simulink model "fv_sim_linearized"  (R2021b)
settings: Solver=VariableStepAuto  StartTime=0.0  StopTime=10  RelTol=1e-3
values from neighbouring files (symbols this model uses):
  euler_angles_BfromN_0_deg = [0.017*0; 0.017*0; 0.017*0]    [run_simulation.m]
  EvB_BfromE_mps = [50; 0.00001; 10]    [run_simulation.m]
  ExE_BfromE_0_m = lla2ecef([lat_d, lon_d, ground_level_m + altitude_m])'    [run_simulation.m]
  g_mps2 = 9.81    [run_simulation.m]
  J_kgm2 = [J_xx, J_xy, J_xz ... (first row only)    [get_mass_props.m]
  ll_NfromE_deg = [lat_d, lon_d]    [run_simulation.m]
  m_kg = sum(cmg(:,1))    [get_mass_props.m]
  omega_BwrtI_rps_0 = omega_BwrtN_rps + omega_EwrtI_rps_0    [run_simulation.m]
  omega_BwrtN_rps = deg2rad(omega_BwrtN_dps)    [run_simulation.m]
  pitch_gain = pitch_kd    [lin_pure_damp.m]    (also in run_simulation.m = -200)
  re_m = 6378000    [run_simulation.m]
  thrust_N = 10    [run_simulation.m]
undefined symbols (not defined in the file or in its folder): aoa_gain, euler_angles_NfromB_0_rad, magnitude, quat_rate_IC
libraries: coordinate_transforms x14, aerolibconvert2 x5, aerolibutil x4, aerolibfltsims x4, simulink_extras x2, vrlib x2, sharedutil x1, aerolibanimutils x1, aerodynamics x1, kinematics x1, slpidlib x1, simulink x1
settings Model: Creator=Nikita  LastModifiedBy=Nikita
settings SolverCC: AlgebraicLoopSolver=TrustRegion
settings DebuggingCC: SFMachineParentedDataDiag=warning

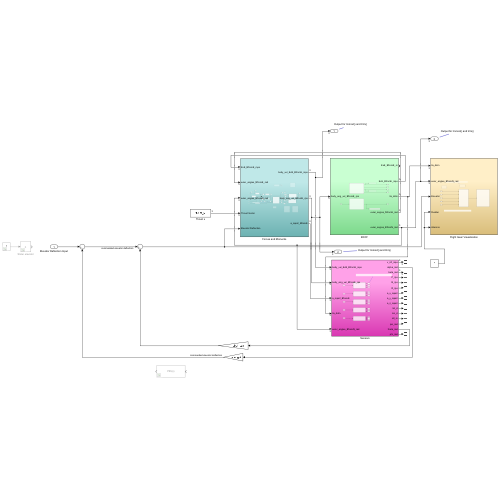
[thumbnail: Simulink's stored preview of the top-level diagram]
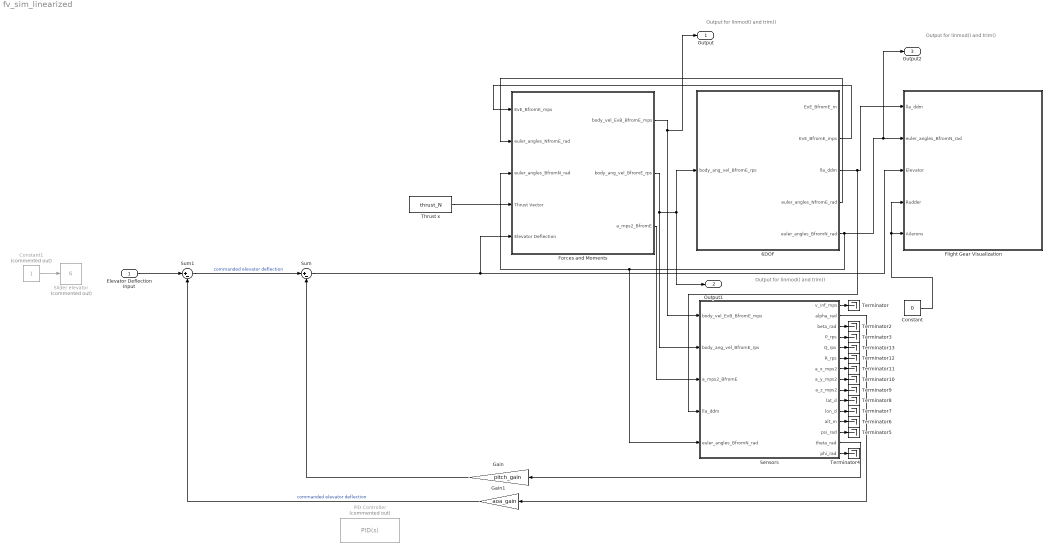
== system fv_sim_linearized ==
  note: Output for linmod() and trim()
  note: Output for linmod() and trim()
  note: Output for linmod() and trim()
  Elevator Deflection Input : Inport
  6DOF : Subsystem
  Constant : Constant  Value=0
  Constant1 : Constant  Commented=on
  Flight Gear Visualization : Subsystem
  Forces and Moments : Subsystem
  Gain : Gain  Gain=pitch_gain
  Gain1 : Gain  Gain=aoa_gain
  PID Controller : slpidlib/PID Controller  Commented=on  Controller=PID  Form=Parallel  TimeDomain=Continuous-time  UseExternalTs=off  SampleTime=-1  IntegratorMethod=Forward Euler  FilterMethod=Forward Euler  ControllerParametersSource=internal  P=-232.326301716838  I=-883.441178625002  D=-13.5750079022675  UseFilter=on  N=74490.174432495  TunerSelectOption=Transfer Function Based (PID Tuner App)  InitialConditionSource=internal  InitialConditionForIntegrator=0  InitialConditionForFilter=0  DifferentiatorICPrevScaledInput=0  ExternalReset=none  TrackingMode=off  Kt=1  LimitOutput=off  SatLimitsSource=internal  UpperSaturationLimit=inf  LowerSaturationLimit=-inf  LinearizeAsGain=on  AntiWindupMode=none  Kb=1  POutMin=[]  POutMax=[]  IOutMin=[]  IOutMax=[]  DOutMin=[]  DOutMax=[]  NOutMin=[]  NOutMax=[]  SumOutMin=[]  SumOutMax=[]  SaturationOutMin=[]  SaturationOutMax=[]  PParamMin=[]  PParamMax=[]  IParamMin=[]  IParamMax=[]  DParamMin=[]  DParamMax=[]  NParamMin=[]  NParamMax=[]  KbParamMin=[]  KbParamMax=[]  KtParamMin=[]  KtParamMax=[]  KbOutMin=[]  KbOutMax=[]  KtOutMin=[]  KtOutMax=[]  IntegratorOutMin=[]  IntegratorOutMax=[]  FilterOutMin=[]  FilterOutMax=[]  SumI1OutMin=[]  SumI1OutMax=[]  SumI2OutMin=[]  SumI2OutMax=[]  SumI3OutMin=[]  SumI3OutMax=[]  SumI4OutMin=[]  SumI4OutMax=[]  SumDOutMin=[]  SumDOutMax=[]  DifferentiatorOutMin=[]  DifferentiatorOutMax=[]  FilterDiffOutCoefMin=[]  FilterDiffOutCoefMax=[]  ReciprocalOutMin=[]  ReciprocalOutMax=[]  SumDenOutMin=[]  SumDenOutMax=[]  SumNumOutMin=[]  SumNumOutMax=[]  DivideOutMin=[]  DivideOutMax=[]  UdiffTsProdOutMin=[]  UdiffTsProdOutMax=[]  NTsProdOutMin=[]  NTsProdOutMax=[]  UintegralTsProdOutMin=[]  UintegralTsProdOutMax=[]  UngainTsProdOutMin=[]  UngainTsProdOutMax=[]  IntegratorContinuousStateAttributes=''  IntegratorStateMustResolveToSignalObject=off  IntegratorRTWStateStorageClass=Auto  FilterContinuousStateAttributes=''  FilterStateMustResolveToSignalObject=off  FilterRTWStateStorageClass=Auto  ParallelPVariant=InternalParameters  IdealPVariant=Disabled  IVariant=InternalParameters  DVariant=InternalParameters  IntegratorVariant=Continuous  SatVariant=Disabled  AWVariant=Passthrough  PCopyVariant=Disabled  TRVariant=Disabled  FdbkBlocksVariant=Forward  IdealPFdbkVariant=Disabled  SatFdbkVariant=Disabled  DerivativeFilterVariant=ContFilter  NVariant=InternalParameters  NCopyVariant=Disabled  FilterICVariant=InternalICsFilter  IntegratorICVariant=InternalICs  ExternalResetVariant=Disabled  TRSumVariant=Passthrough  SumFdbkVariant=Disabled  SumVariant=Sum_PID  TsampFilterVariant=InternalTs  TsampNgainVariant=Passthrough  TsampIntegralVariant=Passthrough  ExternalSaturationOutDataTypeStr=Inherit: Same as second input
  Sensors : Subsystem
  Slider elevator : simulink/Math Operations/Slider Gain  Commented=on  gain=6  low=-10  high=10
  Sum : Sum  Inputs=|+-
  Sum1 : Sum  Inputs=|+-
  Terminator{,2..13} (13 alike) : Terminator
  Thrust x : Constant  Value=thrust_N
  Output : Outport
  Output1 : Outport  Port=2
  Output2 : Outport  Port=3
  wires:
  6DOF/5(euler_angles_BfromN_rad) -> Sensors/5(euler_angles_BfromN_rad), Forces and Moments/3(euler_angles_BfromN_rad), Output2/1, Flight Gear Visualization/2(euler_angles_BfromN_rad)
  Forces and Moments/1(body_vel_EvB_BfromE_mps) -> Output/1, Sensors/1(body_vel_EvB_BfromE_mps)
  6DOF/3(lla_ddm) -> Flight Gear Visualization/1(lla_ddm), Sensors/4(lla_ddm)
  Constant/1 -> Flight Gear Visualization/5(Ailerons), Flight Gear Visualization/4(Rudder)
  6DOF/4(euler_angles_NfromE_rad) -> Forces and Moments/2(euler_angles_NfromE_rad)
  Forces and Moments/2(body_ang_vel_BfromE_rps) -> Sensors/2(body_ang_vel_BfromE_rps), 6DOF/1(body_ang_vel_BfromE_rps), Output1/1
  Forces and Moments/3(a_mps2_BfromE) -> Sensors/3(a_mps2_BfromE)
  Constant1/1 -> Slider elevator/1
  Sensors/14(theta_rad) -> Gain/1
  Sensors/1(v_inf_mps) -> Terminator/1
  Sensors/2(alpha_rad) -> Gain1/1
  Sensors/3(beta_rad) -> Terminator2/1
  Sensors/4(P_rps) -> Terminator3/1
  Sensors/15(phi_rad) -> Terminator4/1
  Sensors/13(psi_rad) -> Terminator5/1
  Sensors/12(alt_m) -> Terminator6/1
  Sensors/11(lon_d) -> Terminator7/1
  Sensors/10(lat_d) -> Terminator8/1
  Sensors/9(a_z_mps2) -> Terminator9/1
  Sensors/8(a_y_mps2) -> Terminator10/1
  Sensors/7(a_x_mps2) -> Terminator11/1
  Sensors/6(R_rps) -> Terminator12/1
  Sensors/5(Q_rps) -> Terminator13/1
  6DOF/2(EvE_BfromE_mps) -> Forces and Moments/1(EvE_BfromE_mps)
  Sum/1 -> Forces and Moments/5(Elevator Deflection), Flight Gear Visualization/3(Elevator)
  Gain/1 -> Sum/2
  Sum1/1 -> Sum/1  "commanded elevator deflection"
  Elevator Deflection Input/1 -> Sum1/1
  Gain1/1 -> Sum1/2  "commanded elevator deflection"
  Thrust x/1 -> Forces and Moments/4(Thrust Vector)

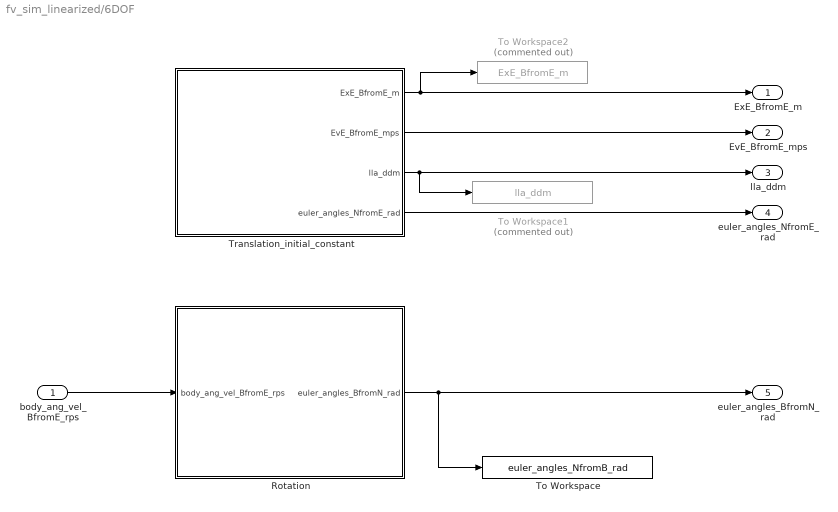
== system fv_sim_linearized/6DOF ==
  body_ang_vel_BfromE_rps : Inport
  Rotation : Subsystem
  To Workspace : ToWorkspace  VariableName=euler_angles_NfromB_rad  SampleTime=-1
  To Workspace1 : ToWorkspace  Commented=on  VariableName=lla_ddm  SampleTime=-1
  To Workspace2 : ToWorkspace  Commented=on  VariableName=ExE_BfromE_m  SampleTime=-1
  Translation_initial_constant : Subsystem
  ExE_BfromE_m : Outport
  EvE_BfromE_mps : Outport  Port=2
  lla_ddm : Outport  Port=3
  euler_angles_NfromE_rad : Outport  Port=4
  euler_angles_BfromN_rad : Outport  Port=5
  wires:
  Translation_initial_constant/3(lla_ddm) -> lla_ddm/1, To Workspace1/1
  Translation_initial_constant/1(ExE_BfromE_m) -> ExE_BfromE_m/1, To Workspace2/1
  Translation_initial_constant/2(EvE_BfromE_mps) -> EvE_BfromE_mps/1
  Rotation/1(euler_angles_BfromN_rad) -> euler_angles_BfromN_rad/1, To Workspace/1
  body_ang_vel_BfromE_rps/1 -> Rotation/1(body_ang_vel_BfromE_rps)
  Translation_initial_constant/4(euler_angles_NfromE_rad) -> euler_angles_NfromE_rad/1

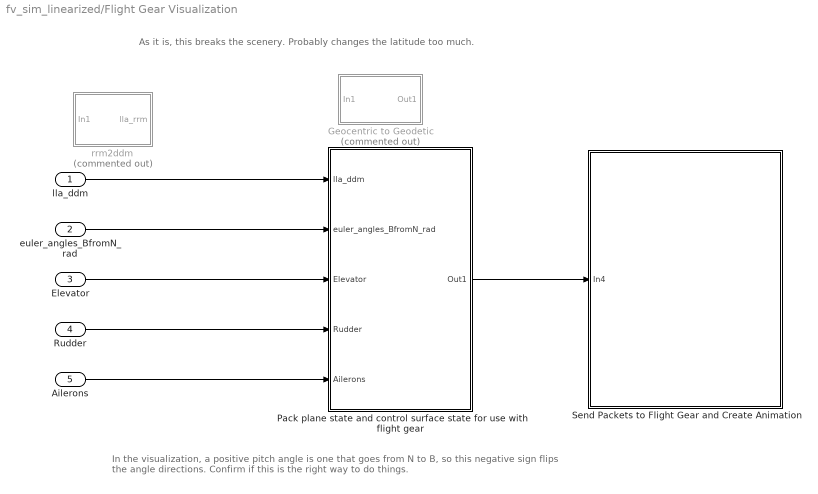
== system fv_sim_linearized/Flight Gear Visualization ==
  note: In the visualization, a positive pitch angle is one that goes from N to B, so this negative sign flips the angle directions. Confirm if this is the right way to do things.
  note: As it is, this breaks the scenery. Probably changes the latitude too much.
  lla_ddm : Inport
  euler_angles_BfromN_rad : Inport  Port=2
  Elevator : Inport  Port=3
  Rudder : Inport  Port=4
  Ailerons : Inport  Port=5
  Geocentric to Geodetic : Subsystem  Commented=on
  Pack plane state and control surface state for use with flight gear : Subsystem
  Send Packets to Flight Gear and Create Animation : Subsystem
  rrm2ddm : Subsystem  Commented=on
  wires:
  lla_ddm/1 -> Pack plane state and control surface state for use with flight gear/1(lla_ddm)
  Elevator/1 -> Pack plane state and control surface state for use with flight gear/3(Elevator)
  Rudder/1 -> Pack plane state and control surface state for use with flight gear/4(Rudder)
  Ailerons/1 -> Pack plane state and control surface state for use with flight gear/5(Ailerons)
  Pack plane state and control surface state for use with flight gear/1(Out1) -> Send Packets to Flight Gear and Create Animation/1(In4)
  euler_angles_BfromN_rad/1 -> Pack plane state and control surface state for use with flight gear/2(euler_angles_BfromN_rad)

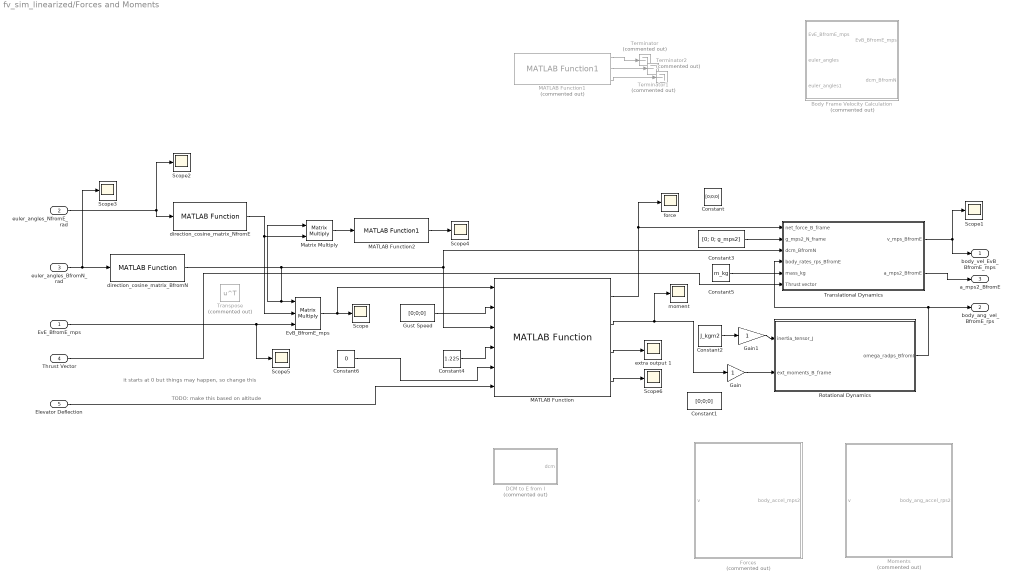
== system fv_sim_linearized/Forces and Moments ==
  note: it starts at 0 but things may happen, so change this
  note: TODO: make this based on altitude
  EvE_BfromE_mps : Inport
  euler_angles_NfromE_rad : Inport  Port=2
  euler_angles_BfromN_rad : Inport  Port=3
  Thrust Vector : Inport  Port=4
  Elevator Deflection : Inport  Port=5
  Body Frame Velocity Calculation : Subsystem  Commented=on
  Constant : Constant  Value=[0;0;0]
  Constant1 : Constant  Value=[0;0;0]
  Constant2 : Constant  Value=J_kgm2
  Constant3 : Constant  Value=[0; 0; g_mps2]
  Constant4 : Constant  Value=1.225
  Constant5 : Constant  Value=m_kg
  Constant6 : Constant  Value=0
  DCM to E from I : Subsystem  Commented=on
  EvB_BfromE_mps : Product  Inputs=3  Multiplication=Matrix(*)
  Forces : Subsystem  Commented=on
  Gain : Gain
  Gain1 : Gain
  Gust Speed : Constant  Value=[0;0;0]
  MATLAB Function : aerodynamics/MATLAB Function  SystemSampleTime=-1  VariantActivationTime=update diagram  Latency=0  AutoFrameSizeCalculation=off
  MATLAB Function1 : kinematics/MATLAB Function1  Commented=on  SystemSampleTime=-1  VariantActivationTime=update diagram  Latency=0  AutoFrameSizeCalculation=off
  MATLAB Function2 : coordinate_transforms/MATLAB Function1  SystemSampleTime=-1  VariantActivationTime=update diagram  Latency=0  AutoFrameSizeCalculation=off
  Matrix Multiply : Product  Multiplication=Matrix(*)
  Moments : Subsystem  Commented=on
  Rotational Dynamics : Subsystem
  Scope{,1..6} (7 alike) : Scope
  Terminator : Terminator  Commented=on
  Terminator1 : Terminator  Commented=on
  Terminator2 : Terminator  Commented=on
  Translational Dynamics : Subsystem
  Transpose : Math  Commented=on  Operator=transpose  SaturateOnIntegerOverflow=on
  direction_cosine_matrix_BfromN : coordinate_transforms/MATLAB Function  SystemSampleTime=-1  VariantActivationTime=update diagram  Latency=0  AutoFrameSizeCalculation=off
  direction_cosine_matrix_NfromE : coordinate_transforms/MATLAB Function  SystemSampleTime=-1  VariantActivationTime=update diagram  Latency=0  AutoFrameSizeCalculation=off
  extra output 1 : Scope
  force : Scope
  moment : Scope
  body_vel_EvB_BfromE_mps : Outport
  body_ang_vel_BfromE_rps : Outport  Port=2
  a_mps2_BfromE : Outport  Port=3
  wires:
  euler_angles_BfromN_rad/1 -> Scope3/1, direction_cosine_matrix_BfromN/1
  Translational Dynamics/1(v_mps_BfromE) -> body_vel_EvB_BfromE_mps/1, Scope1/1
  Rotational Dynamics/1(omega_radps_BfromI) -> body_ang_vel_BfromE_rps/1, Translational Dynamics/4(body_rates_rps_BfromE)
  Constant2/1 -> Gain1/1
  Constant3/1 -> Translational Dynamics/2(g_mps2_N_frame)
  Constant4/1 -> MATLAB Function/4
  Gust Speed/1 -> MATLAB Function/2
  MATLAB Function1/1 -> Terminator/1
  MATLAB Function1/2 -> Terminator1/1
  MATLAB Function1/3 -> Terminator2/1
  Constant5/1 -> Translational Dynamics/5(mass_kg)
  euler_angles_NfromE_rad/1 -> direction_cosine_matrix_NfromE/1, Scope2/1
  direction_cosine_matrix_NfromE/1 -> Matrix Multiply/2, EvB_BfromE_mps/2
  EvE_BfromE_mps/1 -> Scope5/1, EvB_BfromE_mps/3
  EvB_BfromE_mps/1 -> MATLAB Function/1, Scope/1
  MATLAB Function/1 -> force/1, Translational Dynamics/1(net_force_B_frame)
  MATLAB Function/2 -> moment/1, Gain/1
  MATLAB Function/3 -> extra output 1/1
  Gain/1 -> Rotational Dynamics/2(ext_moments_B_frame)
  Gain1/1 -> Rotational Dynamics/1(inertia_tensor_J)
  Constant6/1 -> MATLAB Function/5
  direction_cosine_matrix_BfromN/1 -> EvB_BfromE_mps/1, Matrix Multiply/1, MATLAB Function/3, Translational Dynamics/3(dcm_BfromN)
  MATLAB Function/4 -> Scope6/1
  Matrix Multiply/1 -> MATLAB Function2/1
  MATLAB Function2/1 -> Scope4/1
  Thrust Vector/1 -> Translational Dynamics/6(Thrust vector)
  Translational Dynamics/2(a_mps2_BfromE) -> a_mps2_BfromE/1
  Elevator Deflection/1 -> MATLAB Function/6

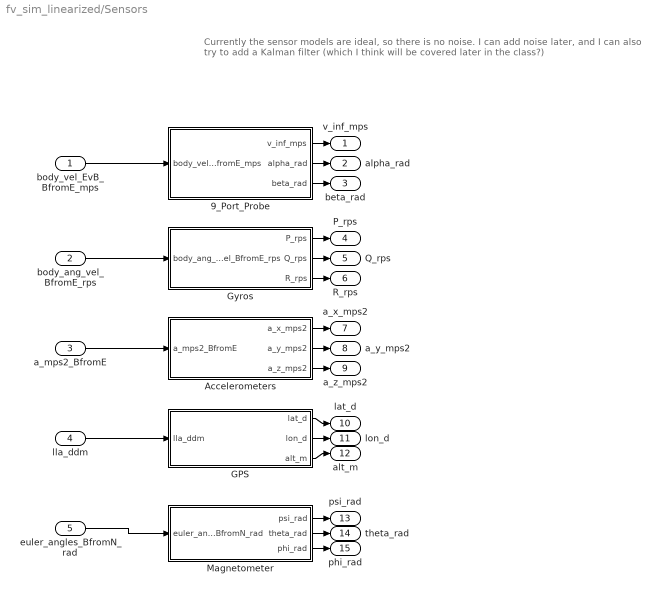
== system fv_sim_linearized/Sensors ==
  note: Currently the sensor models are ideal, so there is no noise. I can add noise later, and I can also try to add a Kalman filter (which I think will be covered later in the class?)
  body_vel_EvB_BfromE_mps : Inport
  body_ang_vel_BfromE_rps : Inport  Port=2
  a_mps2_BfromE : Inport  Port=3
  lla_ddm : Inport  Port=4
  euler_angles_BfromN_rad : Inport  Port=5
  9_Port_Probe : Subsystem
  Accelerometers : Subsystem
  GPS : Subsystem
  Gyros : Subsystem
  Magnetometer : Subsystem
  v_inf_mps : Outport
  alpha_rad : Outport  Port=2
  beta_rad : Outport  Port=3
  P_rps : Outport  Port=4
  Q_rps : Outport  Port=5
  R_rps : Outport  Port=6
  a_x_mps2 : Outport  Port=7
  a_y_mps2 : Outport  Port=8
  a_z_mps2 : Outport  Port=9
  lat_d : Outport  Port=10
  lon_d : Outport  Port=11
  alt_m : Outport  Port=12
  psi_rad : Outport  Port=13
  theta_rad : Outport  Port=14
  phi_rad : Outport  Port=15
  wires:
  9_Port_Probe/3(beta_rad) -> beta_rad/1
  body_vel_EvB_BfromE_mps/1 -> 9_Port_Probe/1(body_vel_EvB_BfromE_mps)
  body_ang_vel_BfromE_rps/1 -> Gyros/1(body_ang_vel_BfromE_rps)
  a_mps2_BfromE/1 -> Accelerometers/1(a_mps2_BfromE)
  Accelerometers/1(a_x_mps2) -> a_x_mps2/1
  Accelerometers/2(a_y_mps2) -> a_y_mps2/1
  9_Port_Probe/1(v_inf_mps) -> v_inf_mps/1
  9_Port_Probe/2(alpha_rad) -> alpha_rad/1
  Gyros/1(P_rps) -> P_rps/1
  Accelerometers/3(a_z_mps2) -> a_z_mps2/1
  Gyros/3(R_rps) -> R_rps/1
  Gyros/2(Q_rps) -> Q_rps/1
  lla_ddm/1 -> GPS/1(lla_ddm)
  GPS/1(lat_d) -> lat_d/1
  GPS/2(lon_d) -> lon_d/1
  GPS/3(alt_m) -> alt_m/1
  euler_angles_BfromN_rad/1 -> Magnetometer/1(euler_angles_BfromN_rad)
  Magnetometer/1(psi_rad) -> psi_rad/1
  Magnetometer/2(theta_rad) -> theta_rad/1
  Magnetometer/3(phi_rad) -> phi_rad/1

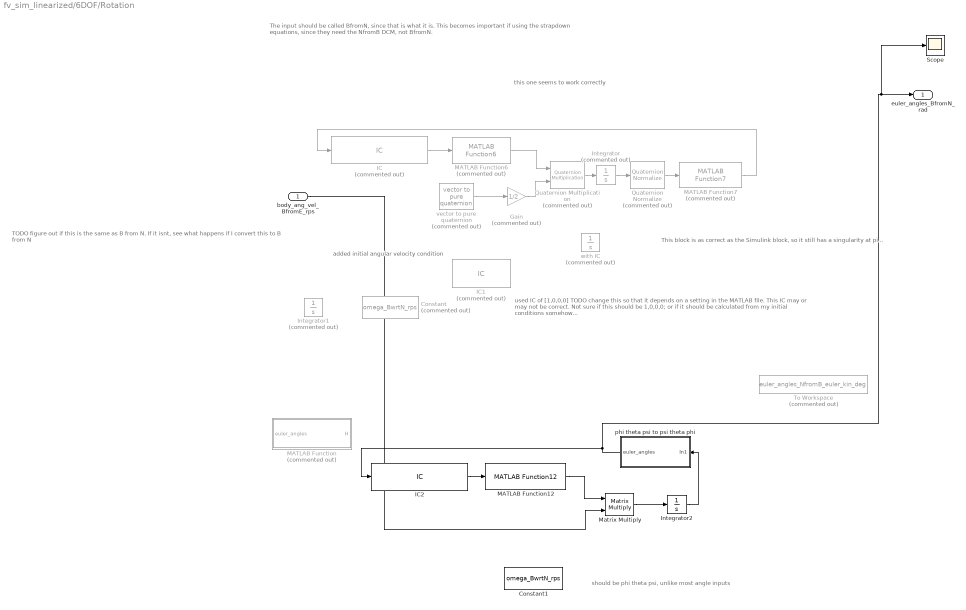
== system fv_sim_linearized/6DOF/Rotation ==
  note: TODO figure out if this is the same as B from N. If it isnt, see what happens if I convert this to B from N
  note: this one seems to work correctly
  note: This block is as correct as the Simulink block, so it still has a singularity at pi...
  note: The input should be called BfromN, since that is what it is.
      |
      | This becomes important if using the strapdown equations, since they need the NfromB DCM, not BfromN.
  note: used IC of [1,0,0,0]
      | TODO change this so that it depends on a setting in the MATLAB file. This IC may or may not be correct.
      | Not sure if this should be 1,0,0,0; or if it should be calculated from my initial conditions somehow...
  note: added initial angular velocity condition
  note: should be phi theta psi, unlike most angle inputs
  body_ang_vel_BfromE_rps : Inport
  Constant : Constant  Commented=on  Value=omega_BwrtN_rps
  Constant1 : Constant  Value=omega_BwrtN_rps
  Gain : Gain  Commented=on  Gain=1/2
  IC : InitialCondition  Commented=on  Value=euler_angles_NfromB_0_rad
  IC1 : InitialCondition  Commented=on  Value=omega_BwrtN_rps
  IC2 : InitialCondition  Value=euler_angles_BfromN_0_deg
  Integrator : Integrator  Commented=on  InitialCondition=[1;0;0;0]
  Integrator1 : Integrator  Commented=on  InitialCondition=omega_BwrtN_rps
  Integrator2 : Integrator  InitialCondition=euler_angles_BfromN_0_deg
  MATLAB Function : MATLAB Function  Commented=on  TreatAsAtomicUnit=on
  MATLAB Function12 : coordinate_transforms/MATLAB Function12  SystemSampleTime=-1  VariantActivationTime=update diagram  Latency=0  AutoFrameSizeCalculation=off
  MATLAB Function6 : coordinate_transforms/MATLAB Function6  Commented=on  SystemSampleTime=-1  VariantActivationTime=update diagram  Latency=0  AutoFrameSizeCalculation=off
  MATLAB Function7 : coordinate_transforms/MATLAB Function7  Commented=on  SystemSampleTime=-1  VariantActivationTime=update diagram  Latency=0  AutoFrameSizeCalculation=off
  Matrix Multiply : Product  Multiplication=Matrix(*)
  Quaternion Multiplication : aerolibutil/Quaternion Multiplication  Commented=on
  Quaternion Normalize : sharedutil/Quaternion Normalize  Commented=on  aMode=aMode
      settings: SourceProductBaseCode=AE,PW,DR,MT,UV,VE
  Scope : Scope
  To Workspace : ToWorkspace  Commented=on  VariableName=euler_angles_NfromB_euler_kin_deg  SampleTime=-1
  phi theta psi to psi theta phi : Subsystem
  vector to pure quaternion : coordinate_transforms/vector to pure quaternion  Commented=on  SystemSampleTime=-1  VariantActivationTime=update diagram  Latency=0  AutoFrameSizeCalculation=off
  with IC : Integrator  Commented=on  InitialCondition=quat_rate_IC
  euler_angles_BfromN_rad : Outport
  wires:
  Quaternion Multiplication/1 -> Integrator/1
  Gain/1 -> Quaternion Multiplication/2
  vector to pure quaternion/1 -> Gain/1
  Integrator/1 -> Quaternion Normalize/1
  IC/1 -> MATLAB Function6/1
  MATLAB Function6/1 -> Quaternion Multiplication/1
  Quaternion Normalize/1 -> MATLAB Function7/1
  MATLAB Function7/1 -> IC/1
  MATLAB Function12/1 -> Matrix Multiply/1
  Matrix Multiply/1 -> Integrator2/1
  Integrator2/1 -> phi theta psi to psi theta phi/1(In1)
  body_ang_vel_BfromE_rps/1 -> Matrix Multiply/2
  phi theta psi to psi theta phi/1(euler_angles) -> Scope/1, euler_angles_BfromN_rad/1, IC2/1
  IC2/1 -> MATLAB Function12/1

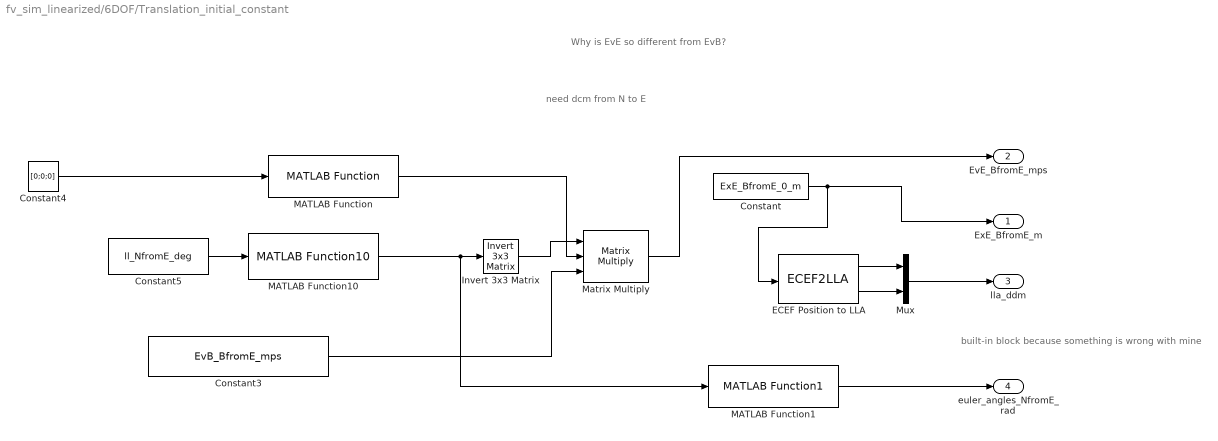
== system fv_sim_linearized/6DOF/Translation_initial_constant ==
  note: Why is EvE so different from EvB?
  note: built-in block because something is wrong with mine
  note: need dcm from N to E
  Constant : Constant  Value=ExE_BfromE_0_m
  Constant3 : Constant  Value=EvB_BfromE_mps
  Constant4 : Constant  Value=[0;0;0]
  Constant5 : Constant  Value=ll_NfromE_deg
  ECEF Position to LLA : ECEF2LLA
  Invert 3x3 Matrix : aerolibutil/Invert  3x3 Matrix
  MATLAB Function : coordinate_transforms/MATLAB Function  SystemSampleTime=-1  VariantActivationTime=update diagram  Latency=0  AutoFrameSizeCalculation=off
  MATLAB Function1 : coordinate_transforms/MATLAB Function1  SystemSampleTime=-1  VariantActivationTime=update diagram  Latency=0  AutoFrameSizeCalculation=off
  MATLAB Function10 : coordinate_transforms/MATLAB Function10  SystemSampleTime=-1  VariantActivationTime=update diagram  Latency=0  AutoFrameSizeCalculation=off
  Matrix Multiply : Product  Inputs=3  Multiplication=Matrix(*)
  Mux : Mux  Inputs=2
  ExE_BfromE_m : Outport
  EvE_BfromE_mps : Outport  Port=2
  lla_ddm : Outport  Port=3
  euler_angles_NfromE_rad : Outport  Port=4
  wires:
  Invert 3x3 Matrix/1 -> Matrix Multiply/1
  Matrix Multiply/1 -> EvE_BfromE_mps/1
  Constant5/1 -> MATLAB Function10/1
  MATLAB Function10/1 -> Invert 3x3 Matrix/1, MATLAB Function1/1
  MATLAB Function1/1 -> euler_angles_NfromE_rad/1
  Constant4/1 -> MATLAB Function/1
  Constant3/1 -> Matrix Multiply/3
  ECEF Position to LLA/2 -> Mux/2
  Mux/1 -> lla_ddm/1
  ECEF Position to LLA/1 -> Mux/1
  MATLAB Function/1 -> Matrix Multiply/2
  Constant/1 -> ECEF Position to LLA/1, ExE_BfromE_m/1

== system fv_sim_linearized/Flight Gear Visualization/Geocentric to Geodetic ==
  In1 : Inport
  Constant1 : Constant  Value=re_m
  Demux : Demux  Outputs=3
  Geocentric to Geodetic Latitude : Geoc2Geod
  Mux2 : Mux  Inputs=3
  Sum : Sum  Inputs=|++
  Out1 : Outport
  wires:
  Constant1/1 -> Sum/2
  Geocentric to Geodetic Latitude/1 -> Mux2/1
  Demux/3 -> Mux2/3, Sum/1
  Demux/1 -> Geocentric to Geodetic Latitude/1
  Sum/1 -> Geocentric to Geodetic Latitude/2
  Demux/2 -> Mux2/2
  In1/1 -> Demux/1
  Mux2/1 -> Out1/1

== system fv_sim_linearized/Flight Gear Visualization/Pack plane state and control surface state for use with flight gear ==
  note: try without this at some point, it seems to change the output data
  note: state (lla_ddm and euler angles in ECEF)
  lla_ddm : Inport
  euler_angles_BfromN_rad : Inport  Port=2
  Elevator : Inport  Port=3
  Rudder : Inport  Port=4
  Ailerons : Inport  Port=5
  Mux : Mux  Inputs=2
  Mux3 : Mux
  Rate Transition : RateTransition  Integrity=off  OutPortSampleTime=1/30
  Out1 : Outport
  wires:
  Ailerons/1 -> Mux3/4
  euler_angles_BfromN_rad/1 -> Mux/2
  Rudder/1 -> Mux3/3
  Mux/1 -> Mux3/1
  Mux3/1 -> Rate Transition/1
  Elevator/1 -> Mux3/2
  Rate Transition/1 -> Out1/1
  lla_ddm/1 -> Mux/1

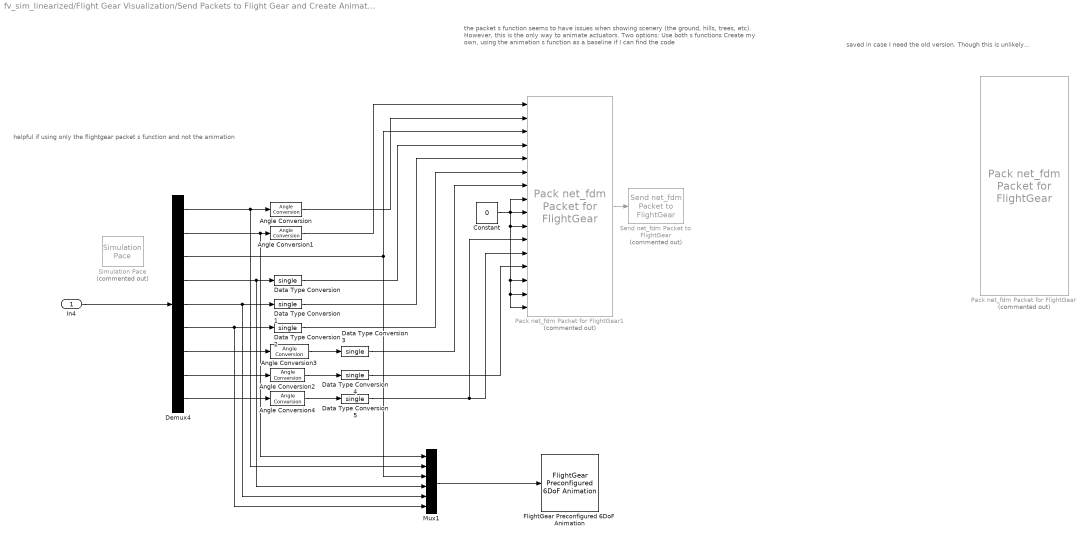
== system fv_sim_linearized/Flight Gear Visualization/Send Packets to Flight Gear and Create Animation ==
  note: the packet s function seems to have issues when showing scenery (the ground, hills, trees, etc). However, this is the only way to animate actuators. Two options:
      | Use both s functions
      | Create my own, using the animation s function as a baseline if I can find the code
  note: saved in case I need the old version. Though this is unlikely...
  note: helpful if using only the flightgear packet s function and not the animation
  In4 : Inport
  Angle Conversion : aerolibconvert2/Angle Conversion  IU=deg  OU=rad
  Angle Conversion1 : aerolibconvert2/Angle Conversion  IU=deg  OU=rad
  Angle Conversion2 : aerolibconvert2/Angle Conversion  IU=rad  OU=deg
  Angle Conversion3 : aerolibconvert2/Angle Conversion  IU=rad  OU=deg
  Angle Conversion4 : aerolibconvert2/Angle Conversion  IU=rad  OU=deg
  Constant : Constant  Value=0
  Data Type Conversion{,1..5} (6 alike) : DataTypeConversion  OutDataTypeStr=single
  Demux4 : Demux  Outputs=9
  FlightGear Preconfigured 6DoF Animation : aerolibfltsims/FlightGear Preconfigured 6DoF Animation  xFlightGearVersion=v2019.1  DestinationIpAddress=127.0.0.1  DestinationPort=5502  SampleTime=1/30  packetVersion=24
  Mux1 : Mux  Inputs=6
  Pack net_fdm Packet for FlightGear : aerolibfltsims/Pack net_fdm Packet for FlightGear  Commented=on  FlightGearVersion=v2019.1  ShowPositionAttitudeInputs=on  ShowVelocityAccelerationInputs=off  ShowControlSurfacePositionInputs=on  ShowEngineFuelInputs=off  ShowLandingGearInputs=off  ShowEnvironmentInputs=off  SampleTime=1/30  packetVersion=24
      settings: SourceProductBaseCode=AE
  Pack net_fdm Packet for FlightGear1 : aerolibfltsims/Pack net_fdm Packet for FlightGear  Commented=on  FlightGearVersion=v2019.1  ShowPositionAttitudeInputs=on  ShowVelocityAccelerationInputs=off  ShowControlSurfacePositionInputs=on  ShowEngineFuelInputs=off  ShowLandingGearInputs=off  ShowEnvironmentInputs=off  SampleTime=1/30  packetVersion=24
      settings: SourceProductBaseCode=AE
  Send net_fdm Packet to FlightGear : aerolibfltsims/Send net_fdm Packet to FlightGear  Commented=on  DestinationIpAddress=127.0.0.1  DestinationPort=5502  LocalIpPort=-1  varLen=off  SampleTime=1/30
      settings: SourceProductBaseCode=AE
  Simulation Pace : aerolibanimutils/Simulation Pace  Commented=on  SimulationPace=1  SleepMode=MATLAB Thread  OutputPaceError=off  SampleTime=1/30
      settings: AttributesFormatString=%<SimulationPace> sec/sec
  wires:
  Data Type Conversion2/1 -> Pack net_fdm Packet for FlightGear1/6
  Mux1/1 -> FlightGear Preconfigured 6DoF Animation/1
  Angle Conversion1/1 -> Pack net_fdm Packet for FlightGear1/1
  Angle Conversion2/1 -> Data Type Conversion4/1
  Demux4/9 -> Angle Conversion4/1
  Angle Conversion3/1 -> Data Type Conversion3/1
  Demux4/3 -> Pack net_fdm Packet for FlightGear1/3, Mux1/3
  Demux4/4 -> Mux1/4, Data Type Conversion/1
  Data Type Conversion5/1 -> Pack net_fdm Packet for FlightGear1/12, Pack net_fdm Packet for FlightGear1/11
  Angle Conversion/1 -> Pack net_fdm Packet for FlightGear1/2
  In4/1 -> Demux4/1
  Demux4/6 -> Mux1/6, Data Type Conversion2/1
  Angle Conversion4/1 -> Data Type Conversion5/1
  Constant/1 -> Pack net_fdm Packet for FlightGear1/9, Pack net_fdm Packet for FlightGear1/8, Pack net_fdm Packet for FlightGear1/16, Pack net_fdm Packet for FlightGear1/15, Pack net_fdm Packet for FlightGear1/14, Pack net_fdm Packet for FlightGear1/10
  Data Type Conversion1/1 -> Pack net_fdm Packet for FlightGear1/5
  Data Type Conversion3/1 -> Pack net_fdm Packet for FlightGear1/7
  Data Type Conversion/1 -> Pack net_fdm Packet for FlightGear1/4
  Demux4/5 -> Mux1/5, Data Type Conversion1/1
  Demux4/1 -> Mux1/2, Angle Conversion/1
  Demux4/2 -> Mux1/1, Angle Conversion1/1
  Demux4/8 -> Angle Conversion2/1
  Data Type Conversion4/1 -> Pack net_fdm Packet for FlightGear1/13
  Demux4/7 -> Angle Conversion3/1
  Pack net_fdm Packet for FlightGear1/1 -> Send net_fdm Packet to FlightGear/1

== system fv_sim_linearized/Flight Gear Visualization/rrm2ddm ==
  In1 : Inport
  Demux : Demux  Outputs=3
  Mux1 : Mux  Inputs=3
  Radians to Degrees : simulink_extras/Transformations/Radians to Degrees
  Radians to Degrees1 : simulink_extras/Transformations/Radians to Degrees
  lla_rrm : Outport
  wires:
  Demux/1 -> Radians to Degrees/1
  Radians to Degrees/1 -> Mux1/1
  Mux1/1 -> lla_rrm/1
  Demux/2 -> Radians to Degrees1/1
  Demux/3 -> Mux1/3
  Radians to Degrees1/1 -> Mux1/2
  In1/1 -> Demux/1

== system fv_sim_linearized/Forces and Moments/Body Frame Velocity Calculation ==
  note: converting EvE velocity to EvB for drag calculation
  EvE_BfromE_mps : Inport
  euler_angles : Inport  Port=2
  euler_angles1 : Inport  Port=3
  Matrix Multiply : Product  Inputs=3  Multiplication=Matrix(*)
  dcm_NfromE : coordinate_transforms/MATLAB Function  SystemSampleTime=-1  VariantActivationTime=update diagram  Latency=0  AutoFrameSizeCalculation=off
  direction_cosine_matrix_BfromN : coordinate_transforms/MATLAB Function  SystemSampleTime=-1  VariantActivationTime=update diagram  Latency=0  AutoFrameSizeCalculation=off
  EvB_BfromE_mps : Outport
  dcm_BfromN : Outport  Port=2
  wires:
  Matrix Multiply/1 -> EvB_BfromE_mps/1
  EvE_BfromE_mps/1 -> Matrix Multiply/3
  direction_cosine_matrix_BfromN/1 -> dcm_BfromN/1, Matrix Multiply/1
  dcm_NfromE/1 -> Matrix Multiply/2
  euler_angles/1 -> direction_cosine_matrix_BfromN/1
  euler_angles1/1 -> dcm_NfromE/1

== system fv_sim_linearized/Forces and Moments/DCM to E from I ==
  note: angles to E from I
  Clock : Clock
  MATLAB Function : coordinate_transforms/MATLAB Function  SystemSampleTime=-1  Latency=0  AutoFrameSizeCalculation=off
  Product : Product
  rotation of Earth : Constant  Value=omega_BwrtI_rps_0
  dcm : Outport
  wires:
  Clock/1 -> Product/1
  Product/1 -> MATLAB Function/1
  rotation of Earth/1 -> Product/2
  MATLAB Function/1 -> dcm/1

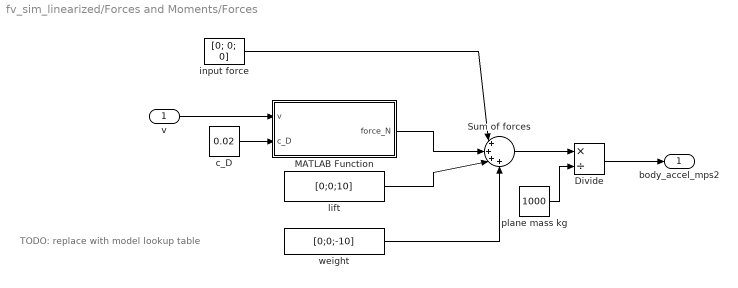
== system fv_sim_linearized/Forces and Moments/Forces ==
  note: TODO: replace with model lookup table
  v : Inport
  Divide : Product  Inputs=*/
  MATLAB Function : MATLAB Function  TreatAsAtomicUnit=on
  Sum of forces : Sum  Inputs=|++++
  c_D : Constant  Value=0.02
  input force : Constant  Value=[0; 0; 0]
  lift : Constant  Value=[0;0;10]
  plane mass kg : Constant  Value=1000
  weight : Constant  Value=[0;0;-10]
  body_accel_mps2 : Outport
  wires:
  input force/1 -> Sum of forces/1
  Divide/1 -> body_accel_mps2/1
  Sum of forces/1 -> Divide/1
  lift/1 -> Sum of forces/3
  MATLAB Function/1(force_N) -> Sum of forces/2
  c_D/1 -> MATLAB Function/2(c_D)
  v/1 -> MATLAB Function/1(v)
  weight/1 -> Sum of forces/4
  plane mass kg/1 -> Divide/2

== system fv_sim_linearized/Forces and Moments/Moments ==
  note: TODO: replace with model lookup table
  v : Inport
  Invert 3x3 Matrix : aerolibutil/Invert  3x3 Matrix
  MATLAB Function1 : MATLAB Function  TreatAsAtomicUnit=on
  Matrix Multiply1 : Product  Multiplication=Matrix(*)
  Sum of moments : Sum  Inputs=|++
  c_m : Constant  Value=0.002
  input moment : Constant  Value=[0; 0; 0]
  plane intertia kgm2 : Constant  Value=[1000,0,0;0,1000,0;0,0,1000]
  body_ang_accel_rps2 : Outport
  wires:
  v/1 -> MATLAB Function1/1(v)
  Sum of moments/1 -> Matrix Multiply1/2
  Invert 3x3 Matrix/1 -> Matrix Multiply1/1
  Matrix Multiply1/1 -> body_ang_accel_rps2/1
  MATLAB Function1/1(body_moment_Nm) -> Sum of moments/2
  plane intertia kgm2/1 -> Invert 3x3 Matrix/1
  input moment/1 -> Sum of moments/1
  c_m/1 -> MATLAB Function1/2(c_m)

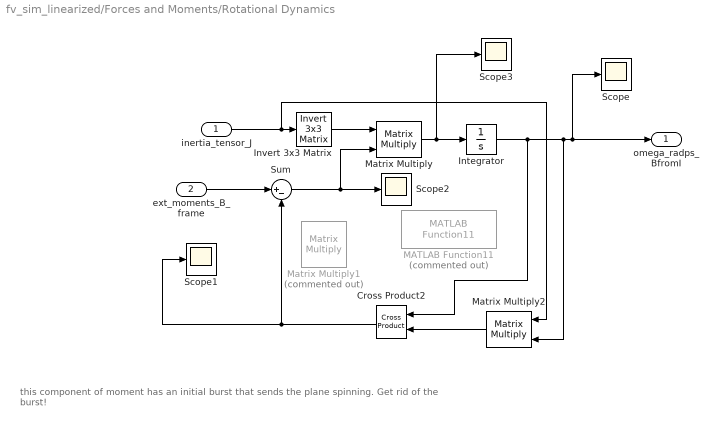
== system fv_sim_linearized/Forces and Moments/Rotational Dynamics ==
  note: this component of moment has an initial burst that sends the plane spinning. Get rid of the burst!
  inertia_tensor_J : Inport
  ext_moments_B_frame : Inport  Port=2
  Cross Product2 : vrlib/Utilities/Cross Product
  Integrator : Integrator  InitialCondition=omega_BwrtI_rps_0
  Invert 3x3 Matrix : aerolibutil/Invert  3x3 Matrix
  MATLAB Function11 : coordinate_transforms/MATLAB Function11  Commented=on  SystemSampleTime=-1  VariantActivationTime=update diagram  Latency=0  AutoFrameSizeCalculation=off
  Matrix Multiply : Product  Multiplication=Matrix(*)
  Matrix Multiply1 : Product  Commented=on  Inputs=3  Multiplication=Matrix(*)
  Matrix Multiply2 : Product  Multiplication=Matrix(*)
  Scope{,1..3} (4 alike) : Scope
  Sum : Sum  Inputs=|+-
  omega_radps_BfromI : Outport
  wires:
  Integrator/1 -> Cross Product2/1, Matrix Multiply2/2, Scope/1, omega_radps_BfromI/1
  inertia_tensor_J/1 -> Matrix Multiply2/1, Invert 3x3 Matrix/1
  Invert 3x3 Matrix/1 -> Matrix Multiply/1
  Sum/1 -> Scope2/1, Matrix Multiply/2
  ext_moments_B_frame/1 -> Sum/1
  Matrix Multiply/1 -> Scope3/1, Integrator/1
  Matrix Multiply2/1 -> Cross Product2/2
  Cross Product2/1 -> Sum/2, Scope1/1

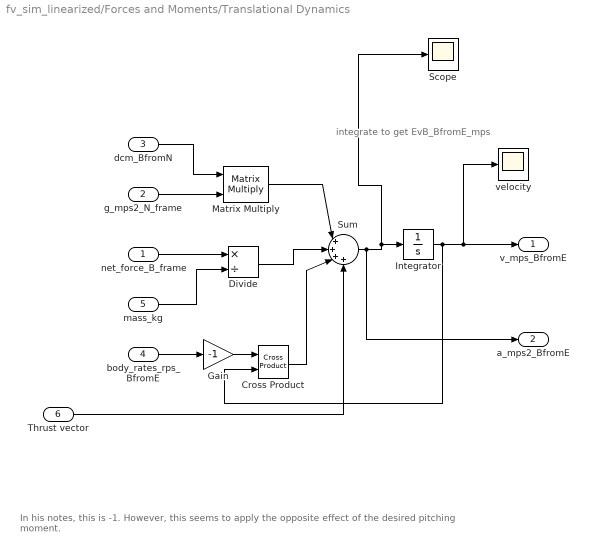
== system fv_sim_linearized/Forces and Moments/Translational Dynamics ==
  note: In his notes, this is -1. However, this seems to apply the opposite effect of the desired pitching moment.
  note: integrate to get EvB_BfromE_mps
  net_force_B_frame : Inport
  g_mps2_N_frame : Inport  Port=2
  dcm_BfromN : Inport  Port=3
  body_rates_rps_BfromE : Inport  Port=4
  mass_kg : Inport  Port=5
  Thrust vector : Inport  Port=6
  Cross Product : vrlib/Utilities/Cross Product
  Divide : Product  Inputs=*/
  Gain : Gain  Gain=-1
  Integrator : Integrator  InitialCondition=EvB_BfromE_mps
  Matrix Multiply : Product  Multiplication=Matrix(*)
  Scope : Scope
  Sum : Sum  Inputs=|++++
  velocity : Scope
  v_mps_BfromE : Outport
  a_mps2_BfromE : Outport  Port=2
  wires:
  g_mps2_N_frame/1 -> Matrix Multiply/2
  dcm_BfromN/1 -> Matrix Multiply/1
  Integrator/1 -> velocity/1, v_mps_BfromE/1, Cross Product/2
  Matrix Multiply/1 -> Sum/1
  net_force_B_frame/1 -> Divide/1
  Sum/1 -> a_mps2_BfromE/1, Scope/1, Integrator/1
  Cross Product/1 -> Sum/3
  body_rates_rps_BfromE/1 -> Gain/1
  Gain/1 -> Cross Product/1
  mass_kg/1 -> Divide/2
  Divide/1 -> Sum/2
  Thrust vector/1 -> Sum/4

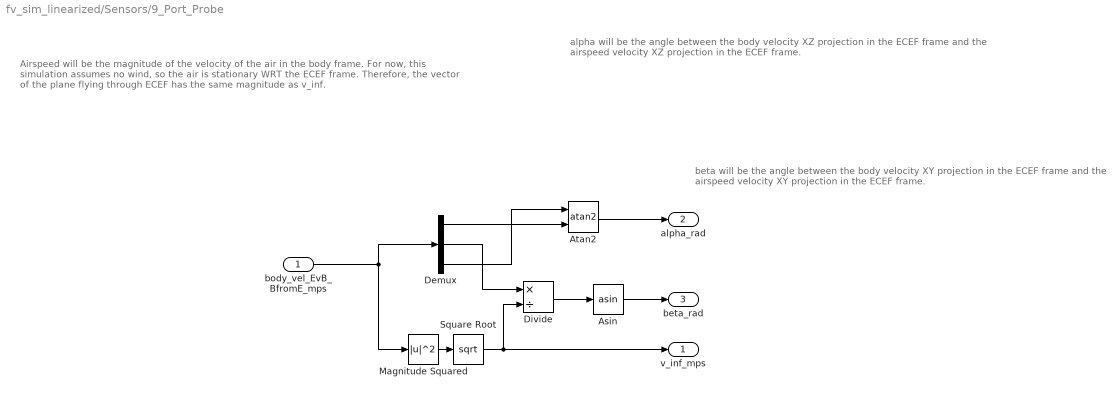
== system fv_sim_linearized/Sensors/9_Port_Probe ==
  note: alpha will be the angle between the body velocity XZ projection in the ECEF frame and the airspeed velocity XZ projection in the ECEF frame.
  note: Airspeed will be the magnitude of the velocity of the air in the body frame. For now, this simulation assumes no wind, so the air is stationary WRT the ECEF frame. Therefore, the vector of the plane flying through ECEF has the same magnitude as v_inf.
  note: beta will be the angle between the body velocity XY projection in the ECEF frame and the airspeed velocity XY projection in the ECEF frame.
  body_vel_EvB_BfromE_mps : Inport
  Asin : Trigonometry  Operator=asin
  Atan2 : Trigonometry  Operator=atan2
  Demux : Demux  Outputs=3
  Divide : Product  Inputs=*/
  Magnitude Squared : Math  Operator=magnitude^2  SaturateOnIntegerOverflow=on
  Square Root : Sqrt  SaturateOnIntegerOverflow=on
  v_inf_mps : Outport
  alpha_rad : Outport  Port=2
  beta_rad : Outport  Port=3
  wires:
  Magnitude Squared/1 -> Square Root/1
  body_vel_EvB_BfromE_mps/1 -> Demux/1, Magnitude Squared/1
  Demux/2 -> Divide/1
  Demux/3 -> Atan2/1
  Square Root/1 -> v_inf_mps/1, Divide/2
  Divide/1 -> Asin/1
  Demux/1 -> Atan2/2
  Asin/1 -> beta_rad/1
  Atan2/1 -> alpha_rad/1

== system fv_sim_linearized/Sensors/Accelerometers ==
  note: Accelerometers measure accelerations in the xyz axes directly. These are in the ECEF frame
  a_mps2_BfromE : Inport
  Demux : Demux  Outputs=3
  a_x_mps2 : Outport
  a_y_mps2 : Outport  Port=2
  a_z_mps2 : Outport  Port=3
  wires:
  Demux/2 -> a_y_mps2/1
  a_mps2_BfromE/1 -> Demux/1
  Demux/1 -> a_x_mps2/1
  Demux/3 -> a_z_mps2/1

== system fv_sim_linearized/Sensors/GPS ==
  note: The GPS receiver gives latitude longitude and altitude in ddm.
  lla_ddm : Inport
  Demux : Demux  Outputs=3
  lat_d : Outport
  lon_d : Outport  Port=2
  alt_m : Outport  Port=3
  wires:
  Demux/3 -> alt_m/1
  Demux/1 -> lat_d/1
  Demux/2 -> lon_d/1
  lla_ddm/1 -> Demux/1

== system fv_sim_linearized/Sensors/Gyros ==
  note: Gyros measure the body rates P, Q, and R
  body_ang_vel_BfromE_rps : Inport
  Demux : Demux  Outputs=3
  P_rps : Outport
  Q_rps : Outport  Port=2
  R_rps : Outport  Port=3
  wires:
  Demux/2 -> Q_rps/1
  Demux/3 -> R_rps/1
  Demux/1 -> P_rps/1
  body_ang_vel_BfromE_rps/1 -> Demux/1

== system fv_sim_linearized/Sensors/Magnetometer ==
  note: This magnetometer is a compass, so it gives yaw angle
  euler_angles_BfromN_rad : Inport
  Demux : Demux  Outputs=3
  psi_rad : Outport
  theta_rad : Outport  Port=2
  phi_rad : Outport  Port=3
  wires:
  euler_angles_BfromN_rad/1 -> Demux/1
  Demux/3 -> phi_rad/1
  Demux/2 -> theta_rad/1
  Demux/1 -> psi_rad/1

== system fv_sim_linearized/6DOF/Rotation/phi theta psi to psi theta phi ==
  In1 : Inport
  Demux : Demux  Outputs=3
  Mux : Mux  Inputs=3
  euler_angles : Outport
  wires:
  Demux/3 -> Mux/1
  In1/1 -> Demux/1
  Demux/1 -> Mux/3
  Demux/2 -> Mux/2
  Mux/1 -> euler_angles/1

== matlab function fv_sim_linearized/Forces and Moments/Forces/MATLAB Function ==
  data: v input; force_N output; c_D input
% Input the velocity vector EvB_BfromE_mps and the total aircraft drag
% coefficient c_D
function force_N = aero_drag(v, c_D)

rho_kgpm3 = 1.225; % TODO replace with a constant
S = 20; % TODO replace with a value from a plane parameter file

% -0.5*r*v^2*S*c_D is scalar. Need to multiply by the v unit vector to get
% direction. norm(v)^2*v/norm(v) = norm(v)*v, therefore:
force_N = -1/2*rho_kgpm3*norm(v)*S*c_D*v;

== matlab function fv_sim_linearized/6DOF/Rotation/MATLAB Function ==
  data: euler_angles input; H output
function H = angles2H(euler_angles)

psi     = euler_angles(1);
theta   = euler_angles(2);
phi     = euler_angles(3);

H = [1,    0,          -sin(theta);
     0, cos(phi),   sin(phi)*cos(theta);
     0, -sin(phi),  cos(phi)*cos(theta)];

== matlab function fv_sim_linearized/Forces and Moments/Moments/MATLAB Function1 ==
  data: v input; body_moment_Nm output; c_m input
% Input the velocity vector EvE_BfromE_mps and the total aircraft pitching
% moment coefficient, c_m
function body_moment_Nm = aero_drag_moment(v, c_m)

rho_kgpm3 = 1.225; % TODO replace with a constant
S = 20; % TODO replace with a value from a plane parameter file
c = 2; % chordlength

j_hat = [0; 1; 0]; % Unit vector in right (Y) direction in the body frame

% 0.5*r*v^2*S*c*c_m is scalar. Need to multiply by the unit vector in the
% right (Y) direction in the body frame.
body_moment_Nm = 1/2*rho_kgpm3*norm(v)^2*S*c*c_m*j_hat;
